simulink model "events_in_stateflow"  (R2018b)
settings: Solver=VariableStepDiscrete  StartTime=0.0  StopTime=10.0  MaxStep=0.5  RelTol=1e-3
settings Model: Creator=marwan  LastModifiedBy=marwan

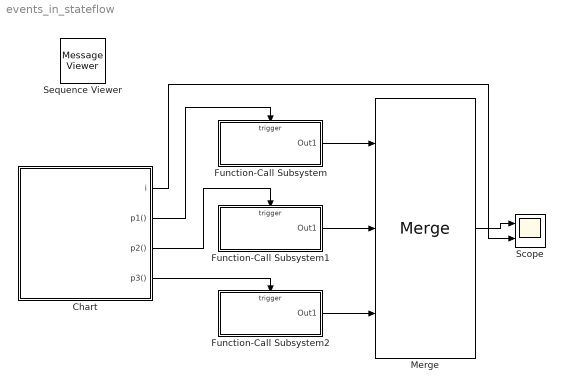
== system events_in_stateflow ==
  Chart : Stateflow chart  TreatAsAtomicUnit=on
  Function-Call Subsystem : Subsystem  TreatAsAtomicUnit=on
  Function-Call Subsystem1 : Subsystem  TreatAsAtomicUnit=on
  Function-Call Subsystem2 : Subsystem  TreatAsAtomicUnit=on
  Merge : Merge  Inputs=3
  Scope : Scope  NumInputPorts=2
  Sequence Viewer : MessageViewer
  wires:
  Chart/2(p1()) -> Function-Call Subsystem/Trigger
  Chart/4(p3()) -> Function-Call Subsystem2/Trigger
  Function-Call Subsystem/1(Out1) -> Merge/1
  Function-Call Subsystem1/1(Out1) -> Merge/2
  Function-Call Subsystem2/1(Out1) -> Merge/3
  Merge/1 -> Scope/1
  Chart/3(p2()) -> Function-Call Subsystem1/Trigger
  Chart/1(i) -> Scope/2

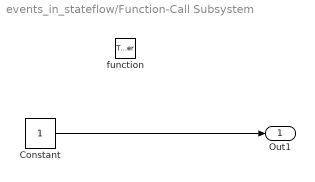
== system events_in_stateflow/Function-Call Subsystem ==
  function : TriggerPort  TriggerType=function-call  VariantControl=Variant
  Constant : Constant
  Out1 : Outport
  wires:
  Constant/1 -> Out1/1

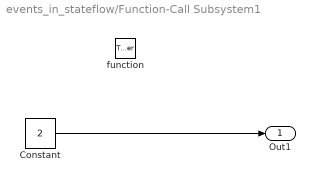
== system events_in_stateflow/Function-Call Subsystem1 ==
  function : TriggerPort  TriggerType=function-call  VariantControl=Variant
  Constant : Constant  Value=2
  Out1 : Outport
  wires:
  Constant/1 -> Out1/1

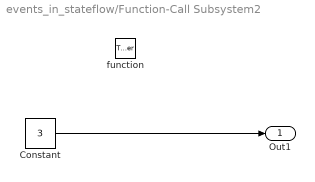
== system events_in_stateflow/Function-Call Subsystem2 ==
  function : TriggerPort  TriggerType=function-call  VariantControl=Variant
  Constant : Constant  Value=3
  Out1 : Outport
  wires:
  Constant/1 -> Out1/1

== stateflow chart events_in_stateflow/Chart ==
  state action [parallel]
    settings: executionOrder=2
    state one
      en: p1;
      du: p1;
    state three
      en: p3;
      du: p3;
    state two
      en: p2;
      du: p2;
    (default) -> one
    three -> one : [i>=3]
    one -> two : [i>=3]
    two -> three : [i>=3]
  state counter [parallel]
    settings: executionOrder=1
    state init
      en: i = 0;
    state count
      en: i = 1;
      du: i = i+1;
    (default) -> init
    init -> count
    count -> count : [i>=3]
  (default) -> action
  data: i output
  events: p1 output FUNCTION_CALL_EVENT; p2 output FUNCTION_CALL_EVENT; p3 output FUNCTION_CALL_EVENT
